simulink model "pendOnlyWithTFim"  (R2019a)
settings: Solver=VariableStepAuto  StartTime=0.0  StopTime=10.0  RelTol=1e-3
undefined symbols (not defined in the file or in its folder): again, Avec1, Avec10, Avec11, Avec2, Avec3, Avec4, Avec5, Avec6, Avec7, Avec8, Avec9, Beq, Bp, Bvec1, Bvec10, Bvec11, Bvec2, Bvec3, Bvec4, Bvec5, Bvec6, Bvec7, Bvec8, Bvec9, Cvec1, Cvec10, Cvec11, Cvec2, Cvec3, Cvec4, Cvec5, Cvec6, Cvec7, Cvec8, Cvec9, Dvec1, Dvec10, Dvec11, Dvec2, Dvec3, Dvec4, Dvec5, Dvec6, Dvec7, Dvec8, Dvec9, Eff_g, Eff_m, g, IMAX_UPM, Ip, Kg, Km, Kt, lp, Mc, Mp, r_mp, Rm ... (+3)
libraries: cstblocks x40, sm_lib x27, nesl_utility x3, simulink_extras x1
(part 2 of 2)

== system pendOnlyWithTFim/Controller/PolesA/Subsystem10/Subsystem4 ==
  In1 : Inport
  DerivativeFilter : cstblocks/LTI System  sys=derivative_filter  IC=[]
  Out1 : Outport
  wires:
  In1/1 -> DerivativeFilter/1
  DerivativeFilter/1 -> Out1/1

== system pendOnlyWithTFim/Controller/PolesA/Subsystem10/Subsystem5 ==
  In1 : Inport
  DerivativeFilter : cstblocks/LTI System  sys=derivative_filter  IC=[]
  Out1 : Outport
  wires:
  In1/1 -> DerivativeFilter/1
  DerivativeFilter/1 -> Out1/1

== system pendOnlyWithTFim/Controller/PolesA/Subsystem10/Subsystem6 ==
  In1 : Inport
  DerivativeFilter : cstblocks/LTI System  sys=derivative_filter  IC=[]
  Out1 : Outport
  wires:
  In1/1 -> DerivativeFilter/1
  DerivativeFilter/1 -> Out1/1

== system pendOnlyWithTFim/Controller/PolesA/Subsystem10/Subsystem7 ==
  In1 : Inport
  DerivativeFilter : cstblocks/LTI System  sys=derivative_filter  IC=[]
  Out1 : Outport
  wires:
  In1/1 -> DerivativeFilter/1
  DerivativeFilter/1 -> Out1/1

== system pendOnlyWithTFim/Controller/PolesA/Subsystem10/Subsystem8 ==
  In1 : Inport
  DerivativeFilter : cstblocks/LTI System  sys=derivative_filter  IC=[]
  Out1 : Outport
  wires:
  In1/1 -> DerivativeFilter/1
  DerivativeFilter/1 -> Out1/1

== system pendOnlyWithTFim/Controller/PolesX/Subsystem10/Subsystem ==
  In1 : Inport
  DerivativeFilter : cstblocks/LTI System  sys=derivative_filter  IC=[]
  Out1 : Outport
  wires:
  In1/1 -> DerivativeFilter/1
  DerivativeFilter/1 -> Out1/1

== system pendOnlyWithTFim/Controller/PolesX/Subsystem10/Subsystem1 ==
  In1 : Inport
  DerivativeFilter : cstblocks/LTI System  sys=derivative_filter  IC=[]
  Out1 : Outport
  wires:
  In1/1 -> DerivativeFilter/1
  DerivativeFilter/1 -> Out1/1

== system pendOnlyWithTFim/Controller/PolesX/Subsystem10/Subsystem10 ==
  In1 : Inport
  DerivativeFilter : cstblocks/LTI System  sys=derivative_filter  IC=[]
  Out1 : Outport
  wires:
  In1/1 -> DerivativeFilter/1
  DerivativeFilter/1 -> Out1/1

== system pendOnlyWithTFim/Controller/PolesX/Subsystem10/Subsystem2 ==
  In1 : Inport
  DerivativeFilter : cstblocks/LTI System  sys=derivative_filter  IC=[]
  Out1 : Outport
  wires:
  In1/1 -> DerivativeFilter/1
  DerivativeFilter/1 -> Out1/1

== system pendOnlyWithTFim/Controller/PolesX/Subsystem10/Subsystem3 ==
  In1 : Inport
  DerivativeFilter : cstblocks/LTI System  sys=derivative_filter  IC=[]
  Out1 : Outport
  wires:
  In1/1 -> DerivativeFilter/1
  DerivativeFilter/1 -> Out1/1

== system pendOnlyWithTFim/Controller/PolesX/Subsystem10/Subsystem4 ==
  In1 : Inport
  DerivativeFilter : cstblocks/LTI System  sys=derivative_filter  IC=[]
  Out1 : Outport
  wires:
  In1/1 -> DerivativeFilter/1
  DerivativeFilter/1 -> Out1/1

== system pendOnlyWithTFim/Controller/PolesX/Subsystem10/Subsystem5 ==
  In1 : Inport
  DerivativeFilter : cstblocks/LTI System  sys=derivative_filter  IC=[]
  Out1 : Outport
  wires:
  In1/1 -> DerivativeFilter/1
  DerivativeFilter/1 -> Out1/1

== system pendOnlyWithTFim/Controller/PolesX/Subsystem10/Subsystem6 ==
  In1 : Inport
  DerivativeFilter : cstblocks/LTI System  sys=derivative_filter  IC=[]
  Out1 : Outport
  wires:
  In1/1 -> DerivativeFilter/1
  DerivativeFilter/1 -> Out1/1

== system pendOnlyWithTFim/Controller/PolesX/Subsystem10/Subsystem7 ==
  In1 : Inport
  DerivativeFilter : cstblocks/LTI System  sys=derivative_filter  IC=[]
  Out1 : Outport
  wires:
  In1/1 -> DerivativeFilter/1
  DerivativeFilter/1 -> Out1/1

== system pendOnlyWithTFim/Controller/PolesX/Subsystem10/Subsystem8 ==
  In1 : Inport
  DerivativeFilter : cstblocks/LTI System  sys=derivative_filter  IC=[]
  Out1 : Outport
  wires:
  In1/1 -> DerivativeFilter/1
  DerivativeFilter/1 -> Out1/1

== system pendOnlyWithTFim/Controller/ZerosA/Subsystem10/Subsystem ==
  In1 : Inport
  DerivativeFilter : cstblocks/LTI System  sys=derivative_filter  IC=[]
  Out1 : Outport
  wires:
  In1/1 -> DerivativeFilter/1
  DerivativeFilter/1 -> Out1/1

== system pendOnlyWithTFim/Controller/ZerosA/Subsystem10/Subsystem1 ==
  In1 : Inport
  DerivativeFilter : cstblocks/LTI System  sys=derivative_filter  IC=[]
  Out1 : Outport
  wires:
  In1/1 -> DerivativeFilter/1
  DerivativeFilter/1 -> Out1/1

== system pendOnlyWithTFim/Controller/ZerosA/Subsystem10/Subsystem10 ==
  In1 : Inport
  DerivativeFilter : cstblocks/LTI System  sys=derivative_filter  IC=[]
  Out1 : Outport
  wires:
  In1/1 -> DerivativeFilter/1
  DerivativeFilter/1 -> Out1/1

== system pendOnlyWithTFim/Controller/ZerosA/Subsystem10/Subsystem2 ==
  In1 : Inport
  DerivativeFilter : cstblocks/LTI System  sys=derivative_filter  IC=[]
  Out1 : Outport
  wires:
  In1/1 -> DerivativeFilter/1
  DerivativeFilter/1 -> Out1/1

== system pendOnlyWithTFim/Controller/ZerosA/Subsystem10/Subsystem3 ==
  In1 : Inport
  DerivativeFilter : cstblocks/LTI System  sys=derivative_filter  IC=[]
  Out1 : Outport
  wires:
  In1/1 -> DerivativeFilter/1
  DerivativeFilter/1 -> Out1/1

== system pendOnlyWithTFim/Controller/ZerosA/Subsystem10/Subsystem4 ==
  In1 : Inport
  DerivativeFilter : cstblocks/LTI System  sys=derivative_filter  IC=[]
  Out1 : Outport
  wires:
  In1/1 -> DerivativeFilter/1
  DerivativeFilter/1 -> Out1/1

== system pendOnlyWithTFim/Controller/ZerosA/Subsystem10/Subsystem5 ==
  In1 : Inport
  DerivativeFilter : cstblocks/LTI System  sys=derivative_filter  IC=[]
  Out1 : Outport
  wires:
  In1/1 -> DerivativeFilter/1
  DerivativeFilter/1 -> Out1/1

== system pendOnlyWithTFim/Controller/ZerosA/Subsystem10/Subsystem6 ==
  In1 : Inport
  DerivativeFilter : cstblocks/LTI System  sys=derivative_filter  IC=[]
  Out1 : Outport
  wires:
  In1/1 -> DerivativeFilter/1
  DerivativeFilter/1 -> Out1/1

== system pendOnlyWithTFim/Controller/ZerosA/Subsystem10/Subsystem7 ==
  In1 : Inport
  DerivativeFilter : cstblocks/LTI System  sys=derivative_filter  IC=[]
  Out1 : Outport
  wires:
  In1/1 -> DerivativeFilter/1
  DerivativeFilter/1 -> Out1/1

== system pendOnlyWithTFim/Controller/ZerosA/Subsystem10/Subsystem8 ==
  In1 : Inport
  DerivativeFilter : cstblocks/LTI System  sys=derivative_filter  IC=[]
  Out1 : Outport
  wires:
  In1/1 -> DerivativeFilter/1
  DerivativeFilter/1 -> Out1/1

== system pendOnlyWithTFim/Controller/ZerosX/Subsystem10/Subsystem ==
  In1 : Inport
  DerivativeFilter : cstblocks/LTI System  sys=derivative_filter  IC=[]
  Out1 : Outport
  wires:
  In1/1 -> DerivativeFilter/1
  DerivativeFilter/1 -> Out1/1

== system pendOnlyWithTFim/Controller/ZerosX/Subsystem10/Subsystem1 ==
  In1 : Inport
  DerivativeFilter : cstblocks/LTI System  sys=derivative_filter  IC=[]
  Out1 : Outport
  wires:
  In1/1 -> DerivativeFilter/1
  DerivativeFilter/1 -> Out1/1

== system pendOnlyWithTFim/Controller/ZerosX/Subsystem10/Subsystem10 ==
  In1 : Inport
  DerivativeFilter : cstblocks/LTI System  sys=derivative_filter  IC=[]
  Out1 : Outport
  wires:
  In1/1 -> DerivativeFilter/1
  DerivativeFilter/1 -> Out1/1

== system pendOnlyWithTFim/Controller/ZerosX/Subsystem10/Subsystem2 ==
  In1 : Inport
  DerivativeFilter : cstblocks/LTI System  sys=derivative_filter  IC=[]
  Out1 : Outport
  wires:
  In1/1 -> DerivativeFilter/1
  DerivativeFilter/1 -> Out1/1

== system pendOnlyWithTFim/Controller/ZerosX/Subsystem10/Subsystem3 ==
  In1 : Inport
  DerivativeFilter : cstblocks/LTI System  sys=derivative_filter  IC=[]
  Out1 : Outport
  wires:
  In1/1 -> DerivativeFilter/1
  DerivativeFilter/1 -> Out1/1

== system pendOnlyWithTFim/Controller/ZerosX/Subsystem10/Subsystem4 ==
  In1 : Inport
  DerivativeFilter : cstblocks/LTI System  sys=derivative_filter  IC=[]
  Out1 : Outport
  wires:
  In1/1 -> DerivativeFilter/1
  DerivativeFilter/1 -> Out1/1

== system pendOnlyWithTFim/Controller/ZerosX/Subsystem10/Subsystem5 ==
  In1 : Inport
  DerivativeFilter : cstblocks/LTI System  sys=derivative_filter  IC=[]
  Out1 : Outport
  wires:
  In1/1 -> DerivativeFilter/1
  DerivativeFilter/1 -> Out1/1

== system pendOnlyWithTFim/Controller/ZerosX/Subsystem10/Subsystem6 ==
  In1 : Inport
  DerivativeFilter : cstblocks/LTI System  sys=derivative_filter  IC=[]
  Out1 : Outport
  wires:
  In1/1 -> DerivativeFilter/1
  DerivativeFilter/1 -> Out1/1

== system pendOnlyWithTFim/Controller/ZerosX/Subsystem10/Subsystem7 ==
  In1 : Inport
  DerivativeFilter : cstblocks/LTI System  sys=derivative_filter  IC=[]
  Out1 : Outport
  wires:
  In1/1 -> DerivativeFilter/1
  DerivativeFilter/1 -> Out1/1

== system pendOnlyWithTFim/Controller/ZerosX/Subsystem10/Subsystem8 ==
  In1 : Inport
  DerivativeFilter : cstblocks/LTI System  sys=derivative_filter  IC=[]
  Out1 : Outport
  wires:
  In1/1 -> DerivativeFilter/1
  DerivativeFilter/1 -> Out1/1

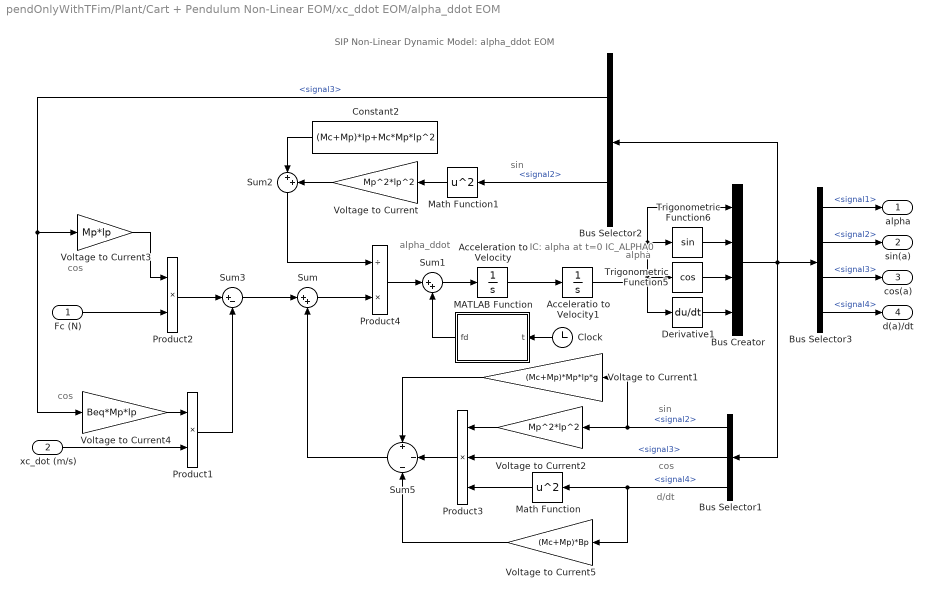
== system pendOnlyWithTFim/Plant/Cart + Pendulum Non-Linear EOM/xc_ddot EOM/alpha_ddot EOM ==
  note: cos
  note: alpha_ddot
  note: IC: alpha at t=0
      | IC_ALPHA0
  note: SIP Non-Linear Dynamic Model:
      | alpha_ddot EOM
  note: alpha
  note: sin
  note: cos
  note: sin
  note: cos
  note: d/dt
  Fc (N) : Inport
  xc_dot (m/s) : Inport  Port=2
  Acceleratio to Velocity1 : Integrator
  Acceleration to Velocity : Integrator
  Bus Creator : BusCreator  Inputs=4
  Bus Selector1 : BusSelector  OutputSignals=signal2,signal3,signal4
  Bus Selector2 : BusSelector  OutputSignals=signal3,signal2
  Bus Selector3 : BusSelector  OutputSignals=signal1,signal2,signal3,signal4
  Clock : Clock
  Constant2 : Constant  Value=(Mc+Mp)*Ip+Mc*Mp*lp^2
  Derivative1 : Derivative
  MATLAB Function : MATLAB Function  TreatAsAtomicUnit=on
  Math Function : Math  Operator=square  SaturateOnIntegerOverflow=on
  Math Function1 : Math  Operator=square  SaturateOnIntegerOverflow=on
  Product1 : Product  SaturateOnIntegerOverflow=on  RndMeth=Zero  InputSameDT=on  OutDataTypeStr=Inherit: Same as first input
  Product2 : Product  SaturateOnIntegerOverflow=on  RndMeth=Zero  InputSameDT=on  OutDataTypeStr=Inherit: Same as first input
  Product3 : Product  Inputs=3  SaturateOnIntegerOverflow=on  RndMeth=Zero  InputSameDT=on  OutDataTypeStr=Inherit: Same as first input
  Product4 : Product  Inputs=/*  SaturateOnIntegerOverflow=on  RndMeth=Zero  InputSameDT=on  OutDataTypeStr=Inherit: Same as first input
  Sum : Sum  Inputs=|++  SaturateOnIntegerOverflow=on  InputSameDT=on  OutDataTypeStr=Inherit: Same as first input
  Sum1 : Sum  Inputs=|++  SaturateOnIntegerOverflow=on  InputSameDT=on  OutDataTypeStr=Inherit: Same as first input
  Sum2 : Sum  Inputs=|++  SaturateOnIntegerOverflow=on  InputSameDT=on  OutDataTypeStr=Inherit: Same as first input
  Sum3 : Sum  Inputs=|+-  SaturateOnIntegerOverflow=on  InputSameDT=on  OutDataTypeStr=Inherit: Same as first input
  Sum5 : Sum  Inputs=+|-|-  SaturateOnIntegerOverflow=on  InputSameDT=on  OutDataTypeStr=Inherit: Same as first input
  Trigonometric Function5 : Trigonometry  Operator=cos
  Trigonometric Function6 : Trigonometry
  Voltage to Current : Gain  Gain=Mp^2*lp^2  SaturateOnIntegerOverflow=on  OutDataTypeStr=Inherit: Same as input  ParamDataTypeStr=Inherit: Same as input
  Voltage to Current1 : Gain  Gain=(Mc+Mp)*Mp*lp*g  SaturateOnIntegerOverflow=on  OutDataTypeStr=Inherit: Same as input  ParamDataTypeStr=Inherit: Same as input
  Voltage to Current2 : Gain  Gain=Mp^2*lp^2  SaturateOnIntegerOverflow=on  OutDataTypeStr=Inherit: Same as input  ParamDataTypeStr=Inherit: Same as input
  Voltage to Current3 : Gain  Gain=Mp*lp  SaturateOnIntegerOverflow=on  OutDataTypeStr=Inherit: Same as input  ParamDataTypeStr=Inherit: Same as input
  Voltage to Current4 : Gain  Gain=Beq*Mp*lp  SaturateOnIntegerOverflow=on  OutDataTypeStr=Inherit: Same as input  ParamDataTypeStr=Inherit: Same as input
  Voltage to Current5 : Gain  Gain=(Mc+Mp)*Bp  SaturateOnIntegerOverflow=on  OutDataTypeStr=Inherit: Same as input  ParamDataTypeStr=Inherit: Same as input
  alpha : Outport  InitialOutput=0
  sin(a) : Outport  Port=2  InitialOutput=0
  cos(a) : Outport  Port=3  InitialOutput=0
  d(a)/dt : Outport  Port=4  InitialOutput=0
  wires:
  Sum5/1 -> Sum/2
  Voltage to Current5/1 -> Sum5/3
  Voltage to Current1/1 -> Sum5/1
  Product3/1 -> Sum5/2
  Sum3/1 -> Sum/1
  Product1/1 -> Sum3/2
  Product2/1 -> Sum3/1
  Voltage to Current4/1 -> Product1/1
  xc_dot (m/s)/1 -> Product1/2
  Fc (N)/1 -> Product2/2
  Voltage to Current3/1 -> Product2/1
  Acceleratio to Velocity1/1 -> Bus Creator/1, Trigonometric Function6/1, Trigonometric Function5/1, Derivative1/1
  Bus Selector3/4 -> d(a)/dt/1  "<signal4>"
  Bus Selector3/3 -> cos(a)/1  "<signal3>"
  Bus Selector3/2 -> sin(a)/1  "<signal2>"
  Bus Selector3/1 -> alpha/1  "<signal1>"
  Bus Selector1/3 -> Voltage to Current5/1, Math Function/1  "<signal4>"
  Bus Selector1/2 -> Product3/2  "<signal3>"
  Voltage to Current2/1 -> Product3/1
  Bus Selector2/1 -> Voltage to Current4/1, Voltage to Current3/1  "<signal3>"
  Bus Creator/1 -> Bus Selector3/1, Bus Selector1/1, Bus Selector2/1
  Derivative1/1 -> Bus Creator/4
  Trigonometric Function5/1 -> Bus Creator/3
  Trigonometric Function6/1 -> Bus Creator/2
  Constant2/1 -> Sum2/1
  Math Function1/1 -> Voltage to Current/1
  Bus Selector2/2 -> Math Function1/1  "<signal2>"
  Voltage to Current/1 -> Sum2/2
  Sum/1 -> Product4/2
  Sum2/1 -> Product4/1
  Math Function/1 -> Product3/3
  Bus Selector1/1 -> Voltage to Current2/1, Voltage to Current1/1  "<signal2>"
  Acceleration to Velocity/1 -> Acceleratio to Velocity1/1
  MATLAB Function/1(fd) -> Sum1/2
  Clock/1 -> MATLAB Function/1(t)
  Product4/1 -> Sum1/1
  Sum1/1 -> Acceleration to Velocity/1

== matlab function pendOnlyWithTFim/Plant/Cart + Pendulum Non-Linear EOM/MATLAB Function ==
  data: t input; fd output
function fd = disturbance(t)
tstart = 2;
tdur = 0.1;
fmag = 0;
if t > tstart && t < tstart + tdur
    fd = fmag;
else
    fd = 0;
end

== matlab function pendOnlyWithTFim/Plant/Cart + Pendulum Non-Linear EOM/xc_ddot EOM/MATLAB Function ==
  data: Fx input; x_dot input; Fstatic output
function Fstatic = fcn(Fx, x_dot)

Fstatic = 0;

x_dot_max2= 0.02;
x_dot_max1 = 0.03;
x_dot_max0 = 0.001;
Fx_max = 1;
b2 = 15;
b1 = 2;

c1 = 1;


if abs(x_dot) < x_dot_max0 && abs(Fx) < Fx_max 
     Fstatic = -Fx;
elseif abs(x_dot) < x_dot_max1 
    Fstatic = -b1*x_dot; %-b1 * x_dot;
else 
    Fstatic = 0;  
end

Fstatic = Fstatic -c1*x_dot*x_dot*sign(x_dot);
end

== matlab function pendOnlyWithTFim/Plant/Cart + Pendulum Non-Linear EOM/xc_ddot EOM/alpha_ddot EOM/MATLAB Function ==
  data: t input; fd output
function fd = disturbance(t)
tstart = 1;
tdur = 0.05;
tend = tstart + tdur;
fmag = 10;
tcycle = 1;
modt = mod(t, tcycle);

if t > tstart && t < tstart + tdur 
    fd = fmag;
else
    fd = 0;
end
end

== matlab function pendOnlyWithTFim/Plant/MATLAB Function ==
  data: v input; x input; v output; theta input
function v = fcn(v,x,theta)

if abs(x) > 0.6|| abs(theta) > 0.6
    v = 0;
end
end
